simulink model "PID_Controller"  (R2020b)
settings: Solver=VariableStepAuto  StartTime=0.0  StopTime=120.0  RelTol=1e-3
settings Model: Creator=Shirish  LastModifiedBy=Shirish
settings DataIOCC: SaveOutput=off  SaveTime=off

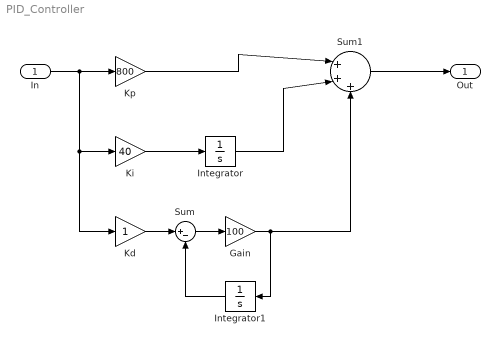
== system PID_Controller ==
  In : Inport  OutDataTypeStr=double  PortDimensions=1  SampleTime=0
  Gain : Gain  Gain=100
  Integrator : Integrator
  Integrator1 : Integrator
  Kd : Gain
  Ki : Gain  Gain=40
  Kp : Gain  Gain=800
  Sum : Sum  Inputs=|+-
  Sum1 : Sum  Inputs=|+++
  Out : Outport  OutDataTypeStr=double  PortDimensions=1  SampleTime=0
  wires:
  Ki/1 -> Integrator/1
  In/1 -> Ki/1, Kd/1, Kp/1
  Kp/1 -> Sum1/1
  Integrator/1 -> Sum1/2
  Sum1/1 -> Out/1
  Gain/1 -> Sum1/3, Integrator1/1
  Integrator1/1 -> Sum/2
  Kd/1 -> Sum/1
  Sum/1 -> Gain/1
